simulink model "QuadcopterModel_PID"  (R2023b)
settings: Solver=VariableStepAuto  StartTime=0.0  StopTime=100  RelTol=1e-3
undefined symbols (not defined in the file): g, Kd_psi, Kd_t, Kd_x, Kd_z, Ki_psi, Ki_t, Ki_x, Ki_z, Kp_psi, Kp_t, Kp_x, Kp_z, m
libraries: slpidlib x6
settings Model: LastModifiedBy=DELL

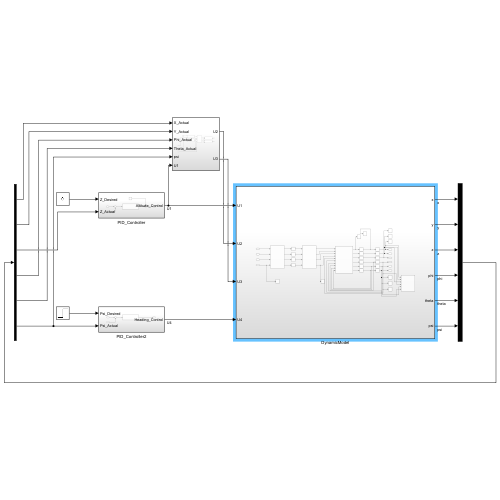
[thumbnail: Simulink's stored preview of the top-level diagram]
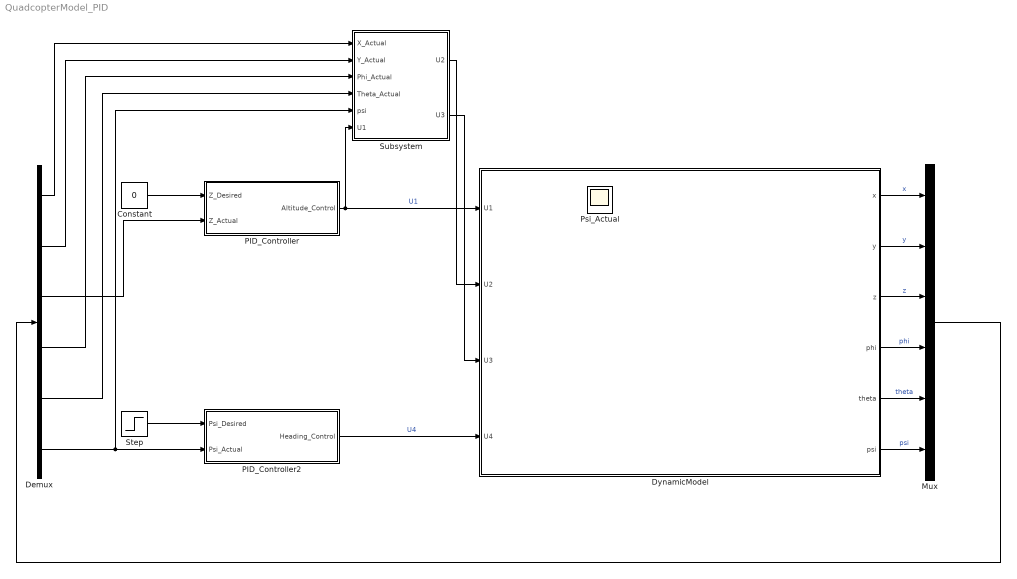
== system QuadcopterModel_PID ==
  Constant : Constant  Value=0
  Demux : Demux  Outputs=6
  DynamicModel : Subsystem
  Mux : Mux  Inputs=6
  PID_Controller : Subsystem
  PID_Controller2 : Subsystem
  Psi_Actual : Scope
  Step : Step  After=0  SampleTime=0
  Subsystem : Subsystem
  wires:
  DynamicModel/3(z) -> Mux/3  "z"
  DynamicModel/5(theta) -> Mux/5  "theta"
  DynamicModel/1(x) -> Mux/1  "x"
  DynamicModel/6(psi) -> Mux/6  "psi"
  DynamicModel/2(y) -> Mux/2  "y"
  DynamicModel/4(phi) -> Mux/4  "phi"
  PID_Controller/1(Altitude_Control) -> Subsystem/6(U1), DynamicModel/1(U1)  "U1"
  Mux/1 -> Demux/1
  Demux/3 -> PID_Controller/2(Z_Actual)
  Constant/1 -> PID_Controller/1(Z_Desired)
  PID_Controller2/1(Heading_Control) -> DynamicModel/4(U4)  "U4"
  Demux/6 -> Subsystem/5(psi), PID_Controller2/2(Psi_Actual)
  Step/1 -> PID_Controller2/1(Psi_Desired)
  Demux/1 -> Subsystem/1(X_Actual)
  Demux/2 -> Subsystem/2(Y_Actual)
  Demux/4 -> Subsystem/3(Phi_Actual)
  Demux/5 -> Subsystem/4(Theta_Actual)
  Subsystem/2(U3) -> DynamicModel/3(U3)
  Subsystem/1(U2) -> DynamicModel/2(U2)

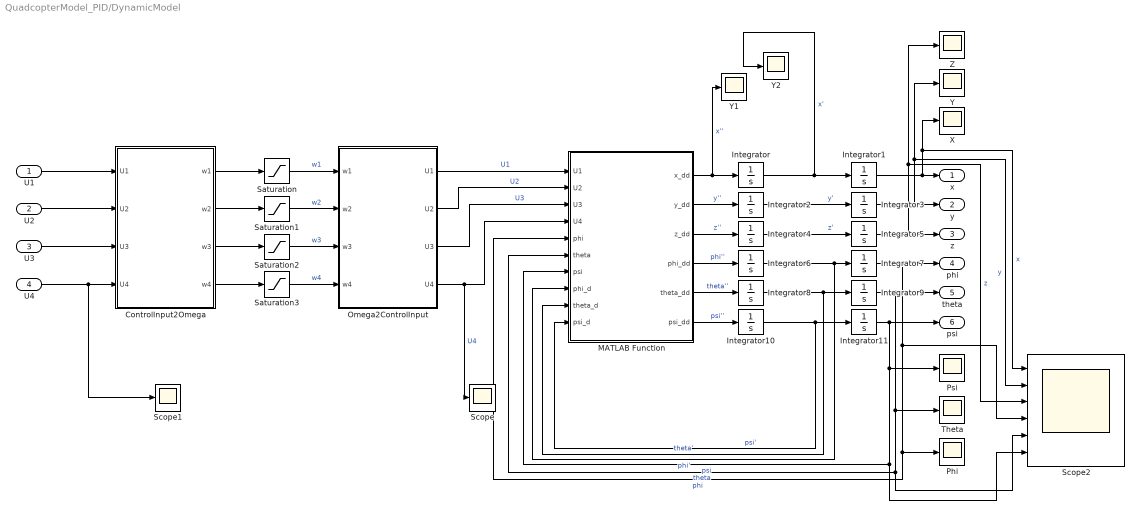
== system QuadcopterModel_PID/DynamicModel ==
  U1 : Inport
  U2 : Inport  Port=2
  U3 : Inport  Port=3
  U4 : Inport  Port=4
  ControlInput2Omega : MATLAB Function  TreatAsAtomicUnit=on
  Integrator{,1..11} (12 alike) : Integrator
  MATLAB Function : MATLAB Function  TreatAsAtomicUnit=on
  Omega2ControlInput : MATLAB Function  TreatAsAtomicUnit=on
  Phi : Scope
  Psi : Scope
  Saturation{,1..3} (4 alike) : Saturate  UpperLimit=550  LowerLimit=0
  Scope : Scope
  Scope1 : Scope
  Scope2 : Scope  NumInputPorts=6
  Theta : Scope
  X : Scope
  Y : Scope
  Y1 : Scope
  Y2 : Scope
  Z : Scope
  x : Outport
  y : Outport  Port=2
  z : Outport  Port=3
  phi : Outport  Port=4
  theta : Outport  Port=5
  psi : Outport  Port=6
  wires:
  Integrator8/1 -> MATLAB Function/9(theta_d), Integrator9/1  "theta'"
  ControlInput2Omega/3(w3) -> Saturation2/1
  Integrator5/1 -> Z/1, Scope2/3, z/1  "z"
  MATLAB Function/1(x_dd) -> Y1/1, Integrator/1  "x''"
  MATLAB Function/5(theta_dd) -> Integrator8/1  "theta''"
  MATLAB Function/6(psi_dd) -> Integrator10/1  "psi''"
  MATLAB Function/3(z_dd) -> Integrator4/1  "z''"
  Saturation2/1 -> Omega2ControlInput/3(w3)  "w3"
  Integrator10/1 -> MATLAB Function/10(psi_d), Integrator11/1  "psi'"
  Integrator6/1 -> MATLAB Function/8(phi_d), Integrator7/1  "phi'"
  MATLAB Function/4(phi_dd) -> Integrator6/1  "phi''"
  Integrator3/1 -> Scope2/2, Y/1, y/1  "y"
  Saturation1/1 -> Omega2ControlInput/2(w2)  "w2"
  ControlInput2Omega/4(w4) -> Saturation3/1
  Integrator4/1 -> Integrator5/1  "z'"
  Saturation/1 -> Omega2ControlInput/1(w1)  "w1"
  Saturation3/1 -> Omega2ControlInput/4(w4)  "w4"
  Integrator11/1 -> psi/1, Scope2/6, MATLAB Function/7(psi), Psi/1  "psi"
  MATLAB Function/2(y_dd) -> Integrator2/1  "y''"
  Integrator2/1 -> Integrator3/1  "y'"
  Integrator7/1 -> phi/1, Scope2/4, MATLAB Function/5(phi), Phi/1  "phi"
  Integrator1/1 -> X/1, Scope2/1, x/1  "x"
  Integrator/1 -> Y2/1, Integrator1/1  "x'"
  ControlInput2Omega/2(w2) -> Saturation1/1
  Integrator9/1 -> Scope2/5, MATLAB Function/6(theta), Theta/1, theta/1  "theta"
  ControlInput2Omega/1(w1) -> Saturation/1
  Omega2ControlInput/2(U2) -> MATLAB Function/2(U2)  "U2"
  U4/1 -> Scope1/1, ControlInput2Omega/4(U4)
  U3/1 -> ControlInput2Omega/3(U3)
  U2/1 -> ControlInput2Omega/2(U2)
  U1/1 -> ControlInput2Omega/1(U1)
  Omega2ControlInput/1(U1) -> MATLAB Function/1(U1)  "U1"
  Omega2ControlInput/3(U3) -> MATLAB Function/3(U3)  "U3"
  Omega2ControlInput/4(U4) -> Scope/1, MATLAB Function/4(U4)  "U4"

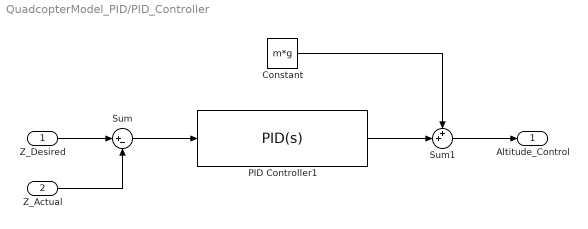
== system QuadcopterModel_PID/PID_Controller ==
  Z_Desired : Inport
  Z_Actual : Inport  Port=2
  Constant : Constant  Value=m*g
  PID Controller1 : slpidlib/PID Controller  Controller=PID  Form=Parallel  TimeDomain=Continuous-time  UseExternalTs=off  SampleTime=-1  IntegratorMethod=Forward Euler  FilterMethod=Forward Euler  ControllerParametersSource=internal  P=Kp_z  I=Ki_z  UseKiTs=off  D=Kd_z  N=100  UseFilter=on  TunerSelectOption=Transfer Function Based (PID Tuner App)  InitialConditionSource=internal  InitialConditionForIntegrator=0  InitialConditionForFilter=0  DifferentiatorICPrevScaledInput=0  ExternalReset=none  TrackingMode=off  Kt=1  LimitOutput=off  SatLimitsSource=internal  UpperSaturationLimit=inf  LowerSaturationLimit=-inf  LinearizeAsGain=on  AntiWindupMode=none  Kb=1  LimitIntegrator=off  UpperIntegratorSaturationLimit=inf  LowerIntegratorSaturationLimit=-inf  POutMin=[]  POutMax=[]  IOutMin=[]  IOutMax=[]  DOutMin=[]  DOutMax=[]  NOutMin=[]  NOutMax=[]  SumOutMin=[]  SumOutMax=[]  SaturationOutMin=[]  SaturationOutMax=[]  PParamMin=[]  PParamMax=[]  IParamMin=[]  IParamMax=[]  DParamMin=[]  DParamMax=[]  NParamMin=[]  NParamMax=[]  KbParamMin=[]  KbParamMax=[]  KtParamMin=[]  KtParamMax=[]  KbOutMin=[]  KbOutMax=[]  KtOutMin=[]  KtOutMax=[]  IntegratorOutMin=[]  IntegratorOutMax=[]  FilterOutMin=[]  FilterOutMax=[]  SumI1OutMin=[]  SumI1OutMax=[]  SumI2OutMin=[]  SumI2OutMax=[]  SumI3OutMin=[]  SumI3OutMax=[]  SumI4OutMin=[]  SumI4OutMax=[]  SumDOutMin=[]  SumDOutMax=[]  DifferentiatorOutMin=[]  DifferentiatorOutMax=[]  FilterDiffOutCoefMin=[]  FilterDiffOutCoefMax=[]  ReciprocalOutMin=[]  ReciprocalOutMax=[]  SumDenOutMin=[]  SumDenOutMax=[]  SumNumOutMin=[]  SumNumOutMax=[]  DivideOutMin=[]  DivideOutMax=[]  UdiffTsProdOutMin=[]  UdiffTsProdOutMax=[]  NTsProdOutMin=[]  NTsProdOutMax=[]  UintegralTsProdOutMin=[]  UintegralTsProdOutMax=[]  UngainTsProdOutMin=[]  UngainTsProdOutMax=[]  ClampingZeroOutDataTypeStr=Inherit: Inherit via back propagation  ClampingZeroOutMin=[]  ClampingZeroOutMax=[]  FilterDenConstantOutDataTypeStr=Inherit: Inherit via back propagation  FilterDenConstantOutMin=[]  FilterDenConstantOutMax=[]  PCopyOutDataTypeStr=Inherit: Inherit via back propagation  PCopyOutMin=[]  PCopyOutMax=[]  NCopyOutDataTypeStr=Inherit: Inherit via back propagation  NCopyOutMin=[]  NCopyOutMax=[]  IntegratorContinuousStateAttributes=''  IntegratorStateMustResolveToSignalObject=off  IntegratorRTWStateStorageClass=Auto  FilterContinuousStateAttributes=''  FilterStateMustResolveToSignalObject=off  FilterRTWStateStorageClass=Auto  ParallelPVariant=InternalParameters  IdealPVariant=Disabled  IVariant=InternalParameters  DVariant=InternalParameters  IntegratorVariant=Continuous  SatVariant=Disabled  AWVariant=Passthrough  PCopyVariant=Disabled  TRVariant=Disabled  FdbkBlocksVariant=Forward  IdealPFdbkVariant=Disabled  SatFdbkVariant=Disabled  DerivativeFilterVariant=ContFilter  NVariant=InternalParameters  NCopyVariant=Disabled  FilterICVariant=InternalICsFilter  IntegratorICVariant=InternalICs  ExternalResetVariant=Disabled  TRSumVariant=Passthrough  SumFdbkVariant=Disabled  SumVariant=Sum_PID  TsampFilterVariant=InternalTs  TsampNgainVariant=Passthrough  TsampIntegralVariant=Disabled_SignalSpec  ExternalSaturationOutDataTypeStr=Inherit: Same as second input
  Sum : Sum  Inputs=|+-
  Sum1 : Sum  Inputs=++|
  Altitude_Control : Outport
  wires:
  Z_Actual/1 -> Sum/2
  Z_Desired/1 -> Sum/1
  Sum/1 -> PID Controller1/1
  Sum1/1 -> Altitude_Control/1
  PID Controller1/1 -> Sum1/2
  Constant/1 -> Sum1/1

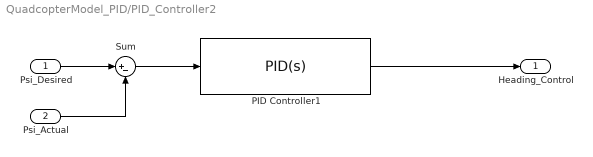
== system QuadcopterModel_PID/PID_Controller2 ==
  Psi_Desired : Inport
  Psi_Actual : Inport  Port=2
  PID Controller1 : slpidlib/PID Controller  Controller=PID  Form=Parallel  TimeDomain=Continuous-time  UseExternalTs=off  SampleTime=-1  IntegratorMethod=Forward Euler  FilterMethod=Forward Euler  ControllerParametersSource=internal  P=Kp_psi  I=Ki_psi  UseKiTs=off  D=Kd_psi  N=100  UseFilter=on  TunerSelectOption=Transfer Function Based (PID Tuner App)  InitialConditionSource=internal  InitialConditionForIntegrator=0  InitialConditionForFilter=0  DifferentiatorICPrevScaledInput=0  ExternalReset=none  TrackingMode=off  Kt=1  LimitOutput=off  SatLimitsSource=internal  UpperSaturationLimit=inf  LowerSaturationLimit=-inf  LinearizeAsGain=on  AntiWindupMode=none  Kb=1  LimitIntegrator=off  UpperIntegratorSaturationLimit=inf  LowerIntegratorSaturationLimit=-inf  POutMin=[]  POutMax=[]  IOutMin=[]  IOutMax=[]  DOutMin=[]  DOutMax=[]  NOutMin=[]  NOutMax=[]  SumOutMin=[]  SumOutMax=[]  SaturationOutMin=[]  SaturationOutMax=[]  PParamMin=[]  PParamMax=[]  IParamMin=[]  IParamMax=[]  DParamMin=[]  DParamMax=[]  NParamMin=[]  NParamMax=[]  KbParamMin=[]  KbParamMax=[]  KtParamMin=[]  KtParamMax=[]  KbOutMin=[]  KbOutMax=[]  KtOutMin=[]  KtOutMax=[]  IntegratorOutMin=[]  IntegratorOutMax=[]  FilterOutMin=[]  FilterOutMax=[]  SumI1OutMin=[]  SumI1OutMax=[]  SumI2OutMin=[]  SumI2OutMax=[]  SumI3OutMin=[]  SumI3OutMax=[]  SumI4OutMin=[]  SumI4OutMax=[]  SumDOutMin=[]  SumDOutMax=[]  DifferentiatorOutMin=[]  DifferentiatorOutMax=[]  FilterDiffOutCoefMin=[]  FilterDiffOutCoefMax=[]  ReciprocalOutMin=[]  ReciprocalOutMax=[]  SumDenOutMin=[]  SumDenOutMax=[]  SumNumOutMin=[]  SumNumOutMax=[]  DivideOutMin=[]  DivideOutMax=[]  UdiffTsProdOutMin=[]  UdiffTsProdOutMax=[]  NTsProdOutMin=[]  NTsProdOutMax=[]  UintegralTsProdOutMin=[]  UintegralTsProdOutMax=[]  UngainTsProdOutMin=[]  UngainTsProdOutMax=[]  ClampingZeroOutDataTypeStr=Inherit: Inherit via back propagation  ClampingZeroOutMin=[]  ClampingZeroOutMax=[]  FilterDenConstantOutDataTypeStr=Inherit: Inherit via back propagation  FilterDenConstantOutMin=[]  FilterDenConstantOutMax=[]  PCopyOutDataTypeStr=Inherit: Inherit via back propagation  PCopyOutMin=[]  PCopyOutMax=[]  NCopyOutDataTypeStr=Inherit: Inherit via back propagation  NCopyOutMin=[]  NCopyOutMax=[]  IntegratorContinuousStateAttributes=''  IntegratorStateMustResolveToSignalObject=off  IntegratorRTWStateStorageClass=Auto  FilterContinuousStateAttributes=''  FilterStateMustResolveToSignalObject=off  FilterRTWStateStorageClass=Auto  ParallelPVariant=InternalParameters  IdealPVariant=Disabled  IVariant=InternalParameters  DVariant=InternalParameters  IntegratorVariant=Continuous  SatVariant=Disabled  AWVariant=Passthrough  PCopyVariant=Disabled  TRVariant=Disabled  FdbkBlocksVariant=Forward  IdealPFdbkVariant=Disabled  SatFdbkVariant=Disabled  DerivativeFilterVariant=ContFilter  NVariant=InternalParameters  NCopyVariant=Disabled  FilterICVariant=InternalICsFilter  IntegratorICVariant=InternalICs  ExternalResetVariant=Disabled  TRSumVariant=Passthrough  SumFdbkVariant=Disabled  SumVariant=Sum_PID  TsampFilterVariant=InternalTs  TsampNgainVariant=Passthrough  TsampIntegralVariant=Disabled_SignalSpec  ExternalSaturationOutDataTypeStr=Inherit: Same as second input
  Sum : Sum  Inputs=|+-
  Heading_Control : Outport
  wires:
  Psi_Actual/1 -> Sum/2
  Psi_Desired/1 -> Sum/1
  Sum/1 -> PID Controller1/1
  PID Controller1/1 -> Heading_Control/1

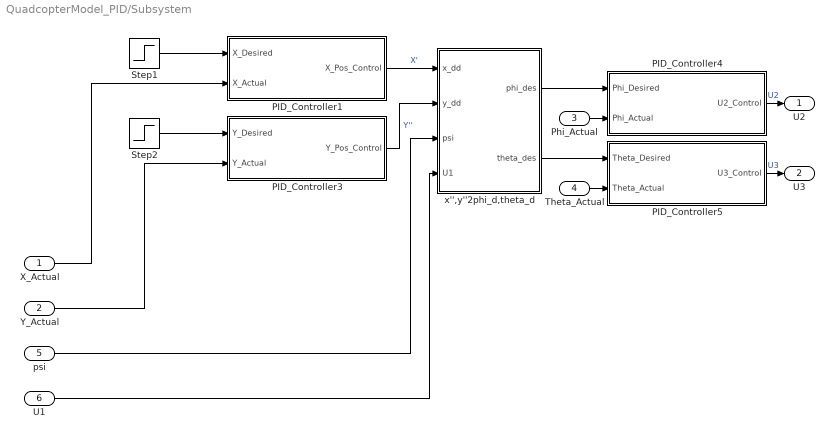
== system QuadcopterModel_PID/Subsystem ==
  X_Actual : Inport
  Y_Actual : Inport  Port=2
  Phi_Actual : Inport  Port=3
  Theta_Actual : Inport  Port=4
  psi : Inport  Port=5
  U1 : Inport  Port=6
  PID_Controller1 : Subsystem
  PID_Controller3 : Subsystem
  PID_Controller4 : Subsystem
  PID_Controller5 : Subsystem
  Step1 : Step  SampleTime=0
  Step2 : Step  After=0  SampleTime=0
  x'',y''2phi_d,theta_d : MATLAB Function  TreatAsAtomicUnit=on
  U2 : Outport
  U3 : Outport  Port=2
  wires:
  Phi_Actual/1 -> PID_Controller4/2(Phi_Actual)
  Y_Actual/1 -> PID_Controller3/2(Y_Actual)
  psi/1 -> x'',y''2phi_d,theta_d/3(psi)
  x'',y''2phi_d,theta_d/2(theta_des) -> PID_Controller5/1(Theta_Desired)
  Step2/1 -> PID_Controller3/1(Y_Desired)
  x'',y''2phi_d,theta_d/1(phi_des) -> PID_Controller4/1(Phi_Desired)
  U1/1 -> x'',y''2phi_d,theta_d/4(U1)
  Step1/1 -> PID_Controller1/1(X_Desired)
  PID_Controller3/1(Y_Pos_Control) -> x'',y''2phi_d,theta_d/2(y_dd)  "Y''"
  Theta_Actual/1 -> PID_Controller5/2(Theta_Actual)
  PID_Controller4/1(U2_Control) -> U2/1  "U2"
  PID_Controller1/1(X_Pos_Control) -> x'',y''2phi_d,theta_d/1(x_dd)  "X'"
  X_Actual/1 -> PID_Controller1/2(X_Actual)
  PID_Controller5/1(U3_Control) -> U3/1  "U3"

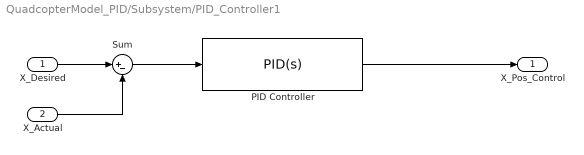
== system QuadcopterModel_PID/Subsystem/PID_Controller1 ==
  X_Desired : Inport
  X_Actual : Inport  Port=2
  PID Controller : slpidlib/PID Controller  Controller=PID  Form=Parallel  TimeDomain=Continuous-time  UseExternalTs=off  SampleTime=-1  IntegratorMethod=Forward Euler  FilterMethod=Forward Euler  ControllerParametersSource=internal  P=Kp_x  I=Ki_x  UseKiTs=off  D=Kd_x  N=100  UseFilter=on  TunerSelectOption=Transfer Function Based (PID Tuner App)  InitialConditionSource=internal  InitialConditionForIntegrator=0  InitialConditionForFilter=0  DifferentiatorICPrevScaledInput=0  ExternalReset=none  TrackingMode=off  Kt=1  LimitOutput=off  SatLimitsSource=internal  UpperSaturationLimit=inf  LowerSaturationLimit=-inf  LinearizeAsGain=on  AntiWindupMode=none  Kb=1  LimitIntegrator=off  UpperIntegratorSaturationLimit=inf  LowerIntegratorSaturationLimit=-inf  POutMin=[]  POutMax=[]  IOutMin=[]  IOutMax=[]  DOutMin=[]  DOutMax=[]  NOutMin=[]  NOutMax=[]  SumOutMin=[]  SumOutMax=[]  SaturationOutMin=[]  SaturationOutMax=[]  PParamMin=[]  PParamMax=[]  IParamMin=[]  IParamMax=[]  DParamMin=[]  DParamMax=[]  NParamMin=[]  NParamMax=[]  KbParamMin=[]  KbParamMax=[]  KtParamMin=[]  KtParamMax=[]  KbOutMin=[]  KbOutMax=[]  KtOutMin=[]  KtOutMax=[]  IntegratorOutMin=[]  IntegratorOutMax=[]  FilterOutMin=[]  FilterOutMax=[]  SumI1OutMin=[]  SumI1OutMax=[]  SumI2OutMin=[]  SumI2OutMax=[]  SumI3OutMin=[]  SumI3OutMax=[]  SumI4OutMin=[]  SumI4OutMax=[]  SumDOutMin=[]  SumDOutMax=[]  DifferentiatorOutMin=[]  DifferentiatorOutMax=[]  FilterDiffOutCoefMin=[]  FilterDiffOutCoefMax=[]  ReciprocalOutMin=[]  ReciprocalOutMax=[]  SumDenOutMin=[]  SumDenOutMax=[]  SumNumOutMin=[]  SumNumOutMax=[]  DivideOutMin=[]  DivideOutMax=[]  UdiffTsProdOutMin=[]  UdiffTsProdOutMax=[]  NTsProdOutMin=[]  NTsProdOutMax=[]  UintegralTsProdOutMin=[]  UintegralTsProdOutMax=[]  UngainTsProdOutMin=[]  UngainTsProdOutMax=[]  ClampingZeroOutDataTypeStr=Inherit: Inherit via back propagation  ClampingZeroOutMin=[]  ClampingZeroOutMax=[]  FilterDenConstantOutDataTypeStr=Inherit: Inherit via back propagation  FilterDenConstantOutMin=[]  FilterDenConstantOutMax=[]  PCopyOutDataTypeStr=Inherit: Inherit via back propagation  PCopyOutMin=[]  PCopyOutMax=[]  NCopyOutDataTypeStr=Inherit: Inherit via back propagation  NCopyOutMin=[]  NCopyOutMax=[]  IntegratorContinuousStateAttributes=''  IntegratorStateMustResolveToSignalObject=off  IntegratorRTWStateStorageClass=Auto  FilterContinuousStateAttributes=''  FilterStateMustResolveToSignalObject=off  FilterRTWStateStorageClass=Auto  ParallelPVariant=InternalParameters  IdealPVariant=Disabled  IVariant=InternalParameters  DVariant=InternalParameters  IntegratorVariant=Continuous  SatVariant=Disabled  AWVariant=Passthrough  PCopyVariant=Disabled  TRVariant=Disabled  FdbkBlocksVariant=Forward  IdealPFdbkVariant=Disabled  SatFdbkVariant=Disabled  DerivativeFilterVariant=ContFilter  NVariant=InternalParameters  NCopyVariant=Disabled  FilterICVariant=InternalICsFilter  IntegratorICVariant=InternalICs  ExternalResetVariant=Disabled  TRSumVariant=Passthrough  SumFdbkVariant=Disabled  SumVariant=Sum_PID  TsampFilterVariant=InternalTs  TsampNgainVariant=Passthrough  TsampIntegralVariant=Disabled_SignalSpec  ExternalSaturationOutDataTypeStr=Inherit: Same as second input
  Sum : Sum  Inputs=|+-
  X_Pos_Control : Outport
  wires:
  X_Actual/1 -> Sum/2
  X_Desired/1 -> Sum/1
  Sum/1 -> PID Controller/1
  PID Controller/1 -> X_Pos_Control/1

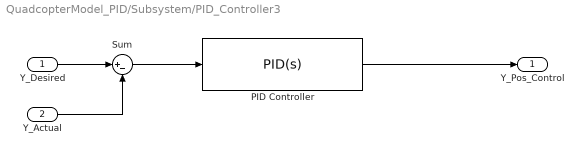
== system QuadcopterModel_PID/Subsystem/PID_Controller3 ==
  Y_Desired : Inport
  Y_Actual : Inport  Port=2
  PID Controller : slpidlib/PID Controller  Controller=PID  Form=Parallel  TimeDomain=Continuous-time  UseExternalTs=off  SampleTime=-1  IntegratorMethod=Forward Euler  FilterMethod=Forward Euler  ControllerParametersSource=internal  P=Kp_x  I=Ki_x  UseKiTs=off  D=Kd_x  N=100  UseFilter=on  TunerSelectOption=Transfer Function Based (PID Tuner App)  InitialConditionSource=internal  InitialConditionForIntegrator=0  InitialConditionForFilter=0  DifferentiatorICPrevScaledInput=0  ExternalReset=none  TrackingMode=off  Kt=1  LimitOutput=off  SatLimitsSource=internal  UpperSaturationLimit=inf  LowerSaturationLimit=-inf  LinearizeAsGain=on  AntiWindupMode=none  Kb=1  LimitIntegrator=off  UpperIntegratorSaturationLimit=inf  LowerIntegratorSaturationLimit=-inf  POutMin=[]  POutMax=[]  IOutMin=[]  IOutMax=[]  DOutMin=[]  DOutMax=[]  NOutMin=[]  NOutMax=[]  SumOutMin=[]  SumOutMax=[]  SaturationOutMin=[]  SaturationOutMax=[]  PParamMin=[]  PParamMax=[]  IParamMin=[]  IParamMax=[]  DParamMin=[]  DParamMax=[]  NParamMin=[]  NParamMax=[]  KbParamMin=[]  KbParamMax=[]  KtParamMin=[]  KtParamMax=[]  KbOutMin=[]  KbOutMax=[]  KtOutMin=[]  KtOutMax=[]  IntegratorOutMin=[]  IntegratorOutMax=[]  FilterOutMin=[]  FilterOutMax=[]  SumI1OutMin=[]  SumI1OutMax=[]  SumI2OutMin=[]  SumI2OutMax=[]  SumI3OutMin=[]  SumI3OutMax=[]  SumI4OutMin=[]  SumI4OutMax=[]  SumDOutMin=[]  SumDOutMax=[]  DifferentiatorOutMin=[]  DifferentiatorOutMax=[]  FilterDiffOutCoefMin=[]  FilterDiffOutCoefMax=[]  ReciprocalOutMin=[]  ReciprocalOutMax=[]  SumDenOutMin=[]  SumDenOutMax=[]  SumNumOutMin=[]  SumNumOutMax=[]  DivideOutMin=[]  DivideOutMax=[]  UdiffTsProdOutMin=[]  UdiffTsProdOutMax=[]  NTsProdOutMin=[]  NTsProdOutMax=[]  UintegralTsProdOutMin=[]  UintegralTsProdOutMax=[]  UngainTsProdOutMin=[]  UngainTsProdOutMax=[]  ClampingZeroOutDataTypeStr=Inherit: Inherit via back propagation  ClampingZeroOutMin=[]  ClampingZeroOutMax=[]  FilterDenConstantOutDataTypeStr=Inherit: Inherit via back propagation  FilterDenConstantOutMin=[]  FilterDenConstantOutMax=[]  PCopyOutDataTypeStr=Inherit: Inherit via back propagation  PCopyOutMin=[]  PCopyOutMax=[]  NCopyOutDataTypeStr=Inherit: Inherit via back propagation  NCopyOutMin=[]  NCopyOutMax=[]  IntegratorContinuousStateAttributes=''  IntegratorStateMustResolveToSignalObject=off  IntegratorRTWStateStorageClass=Auto  FilterContinuousStateAttributes=''  FilterStateMustResolveToSignalObject=off  FilterRTWStateStorageClass=Auto  ParallelPVariant=InternalParameters  IdealPVariant=Disabled  IVariant=InternalParameters  DVariant=InternalParameters  IntegratorVariant=Continuous  SatVariant=Disabled  AWVariant=Passthrough  PCopyVariant=Disabled  TRVariant=Disabled  FdbkBlocksVariant=Forward  IdealPFdbkVariant=Disabled  SatFdbkVariant=Disabled  DerivativeFilterVariant=ContFilter  NVariant=InternalParameters  NCopyVariant=Disabled  FilterICVariant=InternalICsFilter  IntegratorICVariant=InternalICs  ExternalResetVariant=Disabled  TRSumVariant=Passthrough  SumFdbkVariant=Disabled  SumVariant=Sum_PID  TsampFilterVariant=InternalTs  TsampNgainVariant=Passthrough  TsampIntegralVariant=Disabled_SignalSpec  ExternalSaturationOutDataTypeStr=Inherit: Same as second input
  Sum : Sum  Inputs=|+-
  Y_Pos_Control : Outport
  wires:
  Y_Actual/1 -> Sum/2
  Y_Desired/1 -> Sum/1
  Sum/1 -> PID Controller/1
  PID Controller/1 -> Y_Pos_Control/1

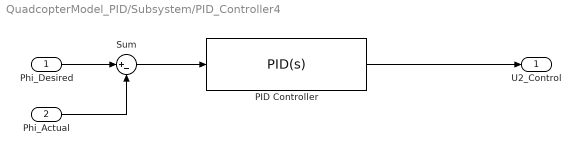
== system QuadcopterModel_PID/Subsystem/PID_Controller4 ==
  Phi_Desired : Inport
  Phi_Actual : Inport  Port=2
  PID Controller : slpidlib/PID Controller  Controller=PID  Form=Parallel  TimeDomain=Continuous-time  UseExternalTs=off  SampleTime=-1  IntegratorMethod=Forward Euler  FilterMethod=Forward Euler  ControllerParametersSource=internal  P=Kp_t  I=Ki_t  UseKiTs=off  D=Kd_t  N=100  UseFilter=on  TunerSelectOption=Transfer Function Based (PID Tuner App)  InitialConditionSource=internal  InitialConditionForIntegrator=0  InitialConditionForFilter=0  DifferentiatorICPrevScaledInput=0  ExternalReset=none  TrackingMode=off  Kt=1  LimitOutput=off  SatLimitsSource=internal  UpperSaturationLimit=inf  LowerSaturationLimit=-inf  LinearizeAsGain=on  AntiWindupMode=none  Kb=1  LimitIntegrator=off  UpperIntegratorSaturationLimit=inf  LowerIntegratorSaturationLimit=-inf  POutMin=[]  POutMax=[]  IOutMin=[]  IOutMax=[]  DOutMin=[]  DOutMax=[]  NOutMin=[]  NOutMax=[]  SumOutMin=[]  SumOutMax=[]  SaturationOutMin=[]  SaturationOutMax=[]  PParamMin=[]  PParamMax=[]  IParamMin=[]  IParamMax=[]  DParamMin=[]  DParamMax=[]  NParamMin=[]  NParamMax=[]  KbParamMin=[]  KbParamMax=[]  KtParamMin=[]  KtParamMax=[]  KbOutMin=[]  KbOutMax=[]  KtOutMin=[]  KtOutMax=[]  IntegratorOutMin=[]  IntegratorOutMax=[]  FilterOutMin=[]  FilterOutMax=[]  SumI1OutMin=[]  SumI1OutMax=[]  SumI2OutMin=[]  SumI2OutMax=[]  SumI3OutMin=[]  SumI3OutMax=[]  SumI4OutMin=[]  SumI4OutMax=[]  SumDOutMin=[]  SumDOutMax=[]  DifferentiatorOutMin=[]  DifferentiatorOutMax=[]  FilterDiffOutCoefMin=[]  FilterDiffOutCoefMax=[]  ReciprocalOutMin=[]  ReciprocalOutMax=[]  SumDenOutMin=[]  SumDenOutMax=[]  SumNumOutMin=[]  SumNumOutMax=[]  DivideOutMin=[]  DivideOutMax=[]  UdiffTsProdOutMin=[]  UdiffTsProdOutMax=[]  NTsProdOutMin=[]  NTsProdOutMax=[]  UintegralTsProdOutMin=[]  UintegralTsProdOutMax=[]  UngainTsProdOutMin=[]  UngainTsProdOutMax=[]  ClampingZeroOutDataTypeStr=Inherit: Inherit via back propagation  ClampingZeroOutMin=[]  ClampingZeroOutMax=[]  FilterDenConstantOutDataTypeStr=Inherit: Inherit via back propagation  FilterDenConstantOutMin=[]  FilterDenConstantOutMax=[]  PCopyOutDataTypeStr=Inherit: Inherit via back propagation  PCopyOutMin=[]  PCopyOutMax=[]  NCopyOutDataTypeStr=Inherit: Inherit via back propagation  NCopyOutMin=[]  NCopyOutMax=[]  IntegratorContinuousStateAttributes=''  IntegratorStateMustResolveToSignalObject=off  IntegratorRTWStateStorageClass=Auto  FilterContinuousStateAttributes=''  FilterStateMustResolveToSignalObject=off  FilterRTWStateStorageClass=Auto  ParallelPVariant=InternalParameters  IdealPVariant=Disabled  IVariant=InternalParameters  DVariant=InternalParameters  IntegratorVariant=Continuous  SatVariant=Disabled  AWVariant=Passthrough  PCopyVariant=Disabled  TRVariant=Disabled  FdbkBlocksVariant=Forward  IdealPFdbkVariant=Disabled  SatFdbkVariant=Disabled  DerivativeFilterVariant=ContFilter  NVariant=InternalParameters  NCopyVariant=Disabled  FilterICVariant=InternalICsFilter  IntegratorICVariant=InternalICs  ExternalResetVariant=Disabled  TRSumVariant=Passthrough  SumFdbkVariant=Disabled  SumVariant=Sum_PID  TsampFilterVariant=InternalTs  TsampNgainVariant=Passthrough  TsampIntegralVariant=Disabled_SignalSpec  ExternalSaturationOutDataTypeStr=Inherit: Same as second input
  Sum : Sum  Inputs=|+-
  U2_Control : Outport
  wires:
  Phi_Actual/1 -> Sum/2
  Phi_Desired/1 -> Sum/1
  Sum/1 -> PID Controller/1
  PID Controller/1 -> U2_Control/1

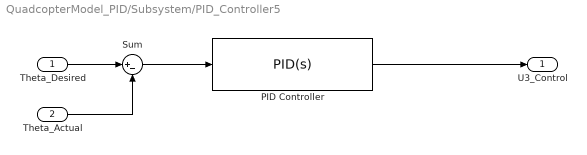
== system QuadcopterModel_PID/Subsystem/PID_Controller5 ==
  Theta_Desired : Inport
  Theta_Actual : Inport  Port=2
  PID Controller : slpidlib/PID Controller  Controller=PID  Form=Parallel  TimeDomain=Continuous-time  UseExternalTs=off  SampleTime=-1  IntegratorMethod=Forward Euler  FilterMethod=Forward Euler  ControllerParametersSource=internal  P=Kp_t  I=Ki_t  UseKiTs=off  D=Kd_t  N=100  UseFilter=on  TunerSelectOption=Transfer Function Based (PID Tuner App)  InitialConditionSource=internal  InitialConditionForIntegrator=0  InitialConditionForFilter=0  DifferentiatorICPrevScaledInput=0  ExternalReset=none  TrackingMode=off  Kt=1  LimitOutput=off  SatLimitsSource=internal  UpperSaturationLimit=inf  LowerSaturationLimit=-inf  LinearizeAsGain=on  AntiWindupMode=none  Kb=1  LimitIntegrator=off  UpperIntegratorSaturationLimit=inf  LowerIntegratorSaturationLimit=-inf  POutMin=[]  POutMax=[]  IOutMin=[]  IOutMax=[]  DOutMin=[]  DOutMax=[]  NOutMin=[]  NOutMax=[]  SumOutMin=[]  SumOutMax=[]  SaturationOutMin=[]  SaturationOutMax=[]  PParamMin=[]  PParamMax=[]  IParamMin=[]  IParamMax=[]  DParamMin=[]  DParamMax=[]  NParamMin=[]  NParamMax=[]  KbParamMin=[]  KbParamMax=[]  KtParamMin=[]  KtParamMax=[]  KbOutMin=[]  KbOutMax=[]  KtOutMin=[]  KtOutMax=[]  IntegratorOutMin=[]  IntegratorOutMax=[]  FilterOutMin=[]  FilterOutMax=[]  SumI1OutMin=[]  SumI1OutMax=[]  SumI2OutMin=[]  SumI2OutMax=[]  SumI3OutMin=[]  SumI3OutMax=[]  SumI4OutMin=[]  SumI4OutMax=[]  SumDOutMin=[]  SumDOutMax=[]  DifferentiatorOutMin=[]  DifferentiatorOutMax=[]  FilterDiffOutCoefMin=[]  FilterDiffOutCoefMax=[]  ReciprocalOutMin=[]  ReciprocalOutMax=[]  SumDenOutMin=[]  SumDenOutMax=[]  SumNumOutMin=[]  SumNumOutMax=[]  DivideOutMin=[]  DivideOutMax=[]  UdiffTsProdOutMin=[]  UdiffTsProdOutMax=[]  NTsProdOutMin=[]  NTsProdOutMax=[]  UintegralTsProdOutMin=[]  UintegralTsProdOutMax=[]  UngainTsProdOutMin=[]  UngainTsProdOutMax=[]  ClampingZeroOutDataTypeStr=Inherit: Inherit via back propagation  ClampingZeroOutMin=[]  ClampingZeroOutMax=[]  FilterDenConstantOutDataTypeStr=Inherit: Inherit via back propagation  FilterDenConstantOutMin=[]  FilterDenConstantOutMax=[]  PCopyOutDataTypeStr=Inherit: Inherit via back propagation  PCopyOutMin=[]  PCopyOutMax=[]  NCopyOutDataTypeStr=Inherit: Inherit via back propagation  NCopyOutMin=[]  NCopyOutMax=[]  IntegratorContinuousStateAttributes=''  IntegratorStateMustResolveToSignalObject=off  IntegratorRTWStateStorageClass=Auto  FilterContinuousStateAttributes=''  FilterStateMustResolveToSignalObject=off  FilterRTWStateStorageClass=Auto  ParallelPVariant=InternalParameters  IdealPVariant=Disabled  IVariant=InternalParameters  DVariant=InternalParameters  IntegratorVariant=Continuous  SatVariant=Disabled  AWVariant=Passthrough  PCopyVariant=Disabled  TRVariant=Disabled  FdbkBlocksVariant=Forward  IdealPFdbkVariant=Disabled  SatFdbkVariant=Disabled  DerivativeFilterVariant=ContFilter  NVariant=InternalParameters  NCopyVariant=Disabled  FilterICVariant=InternalICsFilter  IntegratorICVariant=InternalICs  ExternalResetVariant=Disabled  TRSumVariant=Passthrough  SumFdbkVariant=Disabled  SumVariant=Sum_PID  TsampFilterVariant=InternalTs  TsampNgainVariant=Passthrough  TsampIntegralVariant=Disabled_SignalSpec  ExternalSaturationOutDataTypeStr=Inherit: Same as second input
  Sum : Sum  Inputs=|+-
  U3_Control : Outport
  wires:
  Theta_Actual/1 -> Sum/2
  Theta_Desired/1 -> Sum/1
  Sum/1 -> PID Controller/1
  PID Controller/1 -> U3_Control/1

== matlab function QuadcopterModel_PID/DynamicModel/Omega2ControlInput ==
  data: w1 input; U1 output; w2 input; w3 input; w4 input; U2 output; U3 output; U4 output
function [U1,U2,U3,U4] = fcn(w1,w2,w3,w4)
    
    % COEFFITIENTS
    Kf = 3.13e-5;
    Km = 7.5e-7;

    U1 = Kf * ((w1^2)+(w2^2)+(w3^2)+(w4^2));
    U2 = Kf * (-(w2^2)+(w4^2));
    U3 = Kf * ((w1^2)-(w3^2));
    U4 = Km * ((w1^2)-(w2^2)+(w3^2)-(w4^2));

== matlab function QuadcopterModel_PID/DynamicModel/MATLAB Function ==
  data: U1 input; x_dd output; U2 input; U3 input; U4 input; phi input; theta input; psi input; phi_d input; theta_d input; psi_d input; y_dd output; z_dd output; phi_dd output; theta_dd output; psi_dd output
function [x_dd,y_dd,z_dd,phi_dd,theta_dd,psi_dd] = fcn(U1,U2,U3,U4, phi,theta,psi, phi_d, theta_d, psi_d)
    
    % MOMENTS OF INERTIA
    Ixx = 7.5e-3;
    Iyy = 7.5e-3;
    Izz = 1.3e-2;
    
    % GYRO
    Jr = 0;
    wr = 0;
    
    % LENGTH
    l = 0.23;
    
    % MASS & GRAVITATIONAL ACCELERATION
    m = 0.65;
    %m = 1;
    g = 9.81;
    
    x_dd = -(U1/m)*(sin(phi)*sin(psi)+cos(phi)*cos(psi)*sin(theta));
    y_dd = -(U1/m)*(cos(phi)*sin(psi)*sin(theta)-cos(psi)*sin(phi));
    z_dd = g - (U1/m)*(cos(phi)*cos(theta));

    phi_dd = (l/Ixx)*U2 - (Jr/Ixx)*theta_d*wr + (Iyy/Ixx)*psi_d*theta_d - (Izz/Ixx)*theta_d*psi_d;
    theta_dd = (l/Iyy)*U3 - (Jr/Iyy)*phi_d*wr + (Izz/Iyy)*phi_d*psi_d - (Ixx/Iyy)*psi_d*phi_d;
    psi_dd = (1/Izz)*U4 + (Ixx/Izz)*theta_d*phi_d - (Iyy/Izz)*phi_d*theta_d;

y = [x_dd,y_dd,z_dd,phi_dd,theta_dd,psi_dd];

== matlab function QuadcopterModel_PID/DynamicModel/ControlInput2Omega ==
  data: U1 input; w1 output; U2 input; U3 input; U4 input; w2 output; w3 output; w4 output
function [w1,w2,w3,w4] = fcn(U1,U2,U3,U4)

    % COEFFITIENTS
    Kf = 3.13e-5;
    Km = 7.5e-7;

    w1 = abs((((U1/4)+(U3/2))/Kf + U4/(4*Km)))^(1/2);
    w2 = abs((((U1/4)-(U2/2))/Kf - U4/(4*Km)))^(1/2);
    w3 = abs((((U1/4)-(U3/2))/Kf + U4/(4*Km)))^(1/2);
    w4 = abs((((U1/4)+(U2/2))/Kf - U4/(4*Km)))^(1/2);

    % w1 = sqrt(abs((U1/(4*Kf))+(U3/(2*Kf))+(U4/(4*Km))));
    % w2 = sqrt(abs((U1/(4*Kf))-(U2/(2*Kf))-(U4/(4*Km))));
    % w3 = sqrt(abs((U1/(4*Kf))-(U3/(2*Kf))-(U4/(4*Km))));
    % w4 = sqrt(abs((U1/(4*Kf))+(U2/(2*Kf))-(U4/(4*Km))));

== matlab function QuadcopterModel_PID/Subsystem/x'',y''2phi_d,theta_d ==
  data: phi_des output; theta_des output; x_dd input; y_dd input; psi input; U1 input
function [phi_des,theta_des] = fcn(x_dd,y_dd,psi, U1)
    
    m = 0.65;

    g = (m/U1)*[-sin(psi) cos(psi); -cos(psi) -sin(psi)]*[x_dd;y_dd];

    phi_des = g(1);
    theta_des = g(2);
